simulink model "diff_controller"  (R2024b)
settings: Solver=FixedStepAuto  StartTime=0.0  StopTime=inf  FixedStep=0.001  RelTol=1e-3  EnableMultiTasking=on
InitFcn:
  | Ts = 0.005;
  | diameter = 165; %mm
  | width = 441; %mm
libraries: arduinolib x19, simulink x10, svdutilitieslib x5, simulink_extras x3, arduinosensorlib x2, robotmobilelib x1
(part 2 of 2)

== matlab function diff_controller/Subsystem1/Pose Parser ==
  settings: updateMethod=DISCRETE  sampleTime=Ts
  data: data input; theta output size=[1 1]; distance output size=[1 1]
function [theta, distance] = process_feedback(data)
    % process_feedback searches an array of uint8 values for a valid packet.
    %
    % Packet protocol:
    %   HEADER (uint8)        : 0xAA
    %   THETA (4 x uint8)     : desired theta in rad (stored as 4 bytes)
    %   DISTANCE (4 x uint8)  : desired distance in meter (stored as 4 bytes)
    %   Checksum (uint8)      : XOR checksum of HEADER, THETA, and DISTANCE bytes
    %   Dummy Byte (uint8)    : must equal 0xEE
    %   TERMINATOR (uint8)    : must equal 0xEF
    %
    % If a valid packet is found, the function decodes THETA and DISTANCE;
    % if none is found, it returns the last valid values.
    %
    % The packet is 12 bytes long.
    %

    persistent lastTheta lastDistance;
    if isempty(lastTheta)
        lastTheta = single(0);
    end
    if isempty(lastDistance)
        lastDistance = single(0);
    end

    HEADER   = uint8(170);  % 0xAA
    DUMMY    = uint8(238);  % 0xEE
    TERMINATOR = uint8(239); % 0xEF
    PACKET_SIZE = 12;       

    data = data(:)';

    for i = 1:(length(data) - PACKET_SIZE + 1)
        if data(i) == HEADER
            packet = data(i:(i+PACKET_SIZE-1));

            % Extract fields from the packet:
            % - Byte 1: HEADER (already checked)
            % - Bytes 2-5: THETA bytes
            % - Bytes 6-9: DISTANCE bytes
            % - Byte 10: Checksum
            % - Byte 11: Dummy byte (should equal 0xEE)
            % - Byte 12: Terminator (should equal 0xEF)
            thetaBytes    = packet(2:5);
            distanceBytes = packet(6:9);
            receivedChecksum = packet(10);
            dummy         = packet(11);
            terminator    = packet(12);

            if dummy ~= DUMMY || terminator ~= TERMINATOR
                continue; 
            end
            
            computedChecksum = packet(1);
            for j = 2:9
                computedChecksum = bitxor(computedChecksum, packet(j));
            end

            if computedChecksum ~= receivedChecksum
                continue; 
            end

            theta    = typecast(uint8(thetaBytes), 'single');
            distance = typecast(uint8(distanceBytes), 'single');

            lastTheta = theta;
            lastDistance = distance;
        end
    end

    theta    = lastTheta;
    distance = lastDistance;
   
end

== matlab function diff_controller/Ref Parser/Ref Parser ==
  settings: updateMethod=DISCRETE  sampleTime=Ts
  data: data input; theta output size=[1 1]; distance output size=[1 1]
function [theta, distance] = process_feedback(data)
    % process_feedback searches an array of uint8 values for a valid packet.
    %
    % Packet protocol:
    %   HEADER (uint8)        : 0xAA
    %   THETA (4 x uint8)     : desired theta in rad (stored as 4 bytes)
    %   DISTANCE (4 x uint8)  : desired distance in meter (stored as 4 bytes)
    %   Checksum (uint8)      : XOR checksum of HEADER, THETA, and DISTANCE bytes
    %   Dummy Byte (uint8)    : must equal 0xEE
    %   TERMINATOR (uint8)    : must equal 0xEF
    %
    % If a valid packet is found, the function decodes THETA and DISTANCE;
    % if none is found, it returns the last valid values.
    %
    % The packet is 12 bytes long.
    %

    persistent lastTheta lastDistance;
    if isempty(lastTheta)
        lastTheta = single(0);
    end
    if isempty(lastDistance)
        lastDistance = single(0);
    end

    HEADER   = uint8(170);  % 0xAA
    DUMMY    = uint8(238);  % 0xEE
    TERMINATOR = uint8(239); % 0xEF
    PACKET_SIZE = 12;       

    data = data(:)';

    for i = 1:(length(data) - PACKET_SIZE + 1)
        if data(i) == HEADER
            packet = data(i:(i+PACKET_SIZE-1));

            % Extract fields from the packet:
            % - Byte 1: HEADER (already checked)
            % - Bytes 2-5: THETA bytes
            % - Bytes 6-9: DISTANCE bytes
            % - Byte 10: Checksum
            % - Byte 11: Dummy byte (should equal 0xEE)
            % - Byte 12: Terminator (should equal 0xEF)
            thetaBytes    = packet(2:5);
            distanceBytes = packet(6:9);
            receivedChecksum = packet(10);
            dummy         = packet(11);
            terminator    = packet(12);

            if dummy ~= DUMMY || terminator ~= TERMINATOR
                continue; 
            end
            
            computedChecksum = packet(1);
            for j = 2:9
                computedChecksum = bitxor(computedChecksum, packet(j));
            end

            if computedChecksum ~= receivedChecksum
                continue; 
            end

            theta    = typecast(uint8(thetaBytes), 'single');
            distance = typecast(uint8(distanceBytes), 'single');

            lastTheta = theta;
            lastDistance = distance;
        end
    end

    theta    = lastTheta;
    distance = lastDistance;
   
end

== stateflow chart diff_controller/Chart1 ==
  settings: updateMethod=DISCRETE  sampleTime=Ts
  state Moving
    entry:
    steer_rear = 0;
    speed_rear = 100;
    stear_front = 0;
    speed_front = 0;
    during:
    measured_distance = measured_distance + current_encoder_velocity;
  state Init
    entry:
    steer_rear = 0;
    speed_rear = 0;
    stear_front = 0;
    speed_front = 0;
  state Stopped
    entry:
    steer_rear = 0;
    speed_rear = 0;
    stear_front = 0;
    speed_front = 0;
  state Rotating
    entry:
    steer_rear = 100;
    speed_rear = 0;
    stear_front = -100;
    speed_front = 0;
    during:
    measured_angle = measured_angle + current_angular_velocity;
    exit:
    measured_distance = 0;
    measured_angle = 0;
  (default) -> Init
  Init -> Moving : after(10,sec)
  Stopped -> Moving [order 1] : [measured_distance < set_point]
  Moving -> Stopped : [measured_distance >= set_point]
  Rotating -> Stopped : [measured_angle >= 180]
  Stopped -> Rotating [order 2] : [measured_distance >= set_point]
      | {after(1,sec)}
  data: speed_rear output; current_encoder_velocity input; current_angular_velocity input; set_point input; steer_rear output; measured_distance output =0; speed_front output; stear_front output; measured_angle output =0

== matlab function diff_controller/Encoders/Encoder Parser ==
  settings: updateMethod=DISCRETE  sampleTime=Ts
  data: sample input; rightSpeed output; leftSpeed output
function [rightSpeed, leftSpeed] = encoder_parser(sample)

    persistent rSpeed;
    persistent lSpeed;

    if isempty(rSpeed)
        rSpeed = 0;
        lSpeed = 0;
    end
    headers = find(sample == -21555);
    if diff(headers) == 9
        rSpeed = double(sample(headers(1)+3));
        lSpeed = double(sample(headers(1)+4));
        rightSpeed = -1*rSpeed;
        leftSpeed = lSpeed;
    else
        rightSpeed = -1*rSpeed;
        leftSpeed = lSpeed;
    end
end

== stateflow chart diff_controller/Chart ==
  state Init
    entry:
    steer = 0;
    speed = 0;
  state Moving
    entry:
    steer = 0;
    speed = 100;
  state Rotating
    entry:
    steer = 100;
    speed = 0;
  state Stopped
    entry:
    steer = 0;
    speed = 0;
  (default) -> Init
  Init -> Moving
  Stopped -> Moving [order 1] : [measured_distance < 10 && utrasonic_status == 0]
  Moving -> Stopped : [measured_distance >= 10 || utrasonic_status == 1]
  Rotating -> Stopped : [measured_angle >= 180]
  Stopped -> Rotating [order 2] : [measured_distance >= 10]
  data: utrasonic_status input; measured_distance input; speed output; steer output; measured_angle input

== stateflow chart diff_controller/Chart2 ==
  settings: updateMethod=DISCRETE  sampleTime=Ts
  state Moving
    entry:
    steer_rear = 100;
    speed_rear = 0;
    stear_front =  100;
    speed_front = 0;
    during:
    steer_rear = 100;
    speed_rear = 0;
    stear_front =  100;
    speed_front = 0;
  state Init
    entry:
    steer_rear = 0;
    speed_rear = 0;
    stear_front = 0;
    speed_front = 0;
  (default) -> Init
  Init -> Moving : after(10,sec)
  data: speed_rear output; steer_rear output; speed_front output; stear_front output

== matlab function diff_controller/Encoders1/Encoder Parser ==
  settings: updateMethod=DISCRETE  sampleTime=Ts
  data: sample input; rightSpeed output; leftSpeed output
function [rightSpeed, leftSpeed] = encoder_parser(sample)

    persistent rSpeed;
    persistent lSpeed;

    if isempty(rSpeed)
        rSpeed = 0;
        lSpeed = 0;
    end
    headers = find(sample == -21555);
    if diff(headers) == 9
        rSpeed = double(sample(headers(1)+3));
        lSpeed = double(sample(headers(1)+4));
        rightSpeed = -1*rSpeed;
        leftSpeed = lSpeed;
    else
        rightSpeed = -1*rSpeed;
        leftSpeed = lSpeed;
    end
end

== matlab function diff_controller/Encoders Right/Encoder Parser ==
  settings: updateMethod=DISCRETE  sampleTime=Ts
  data: data input; averageSpeed output
function averageSpeed = process_feedback(data)

% Feedback is sent every 10ms:
% 
% Start frame(unsigned int16) : 0xABCD
% Cmd1(signed int16) : Steer or Brake(hovercar) after normalizing and mixing
% Cmd2(signed int16) : Speed or Throttle(hovercar) after normalizing and mixing
% SpeedR(signed int16) : Measured right wheel speed in RPM
% SpeedL(signed int16) : Measured left wheel speed in RPM
% Battery Voltage(signed int16) : Calibrated Battery Voltage *100
% Temperature(signed int16) : Temperature in °C *10
% Led(unsigned int16) : Used to control the leds on the sideboard
% Checksum(unsigned int16) : XOR checksum
%
%

    persistent lastValidAverageSpeed;

    if isempty(lastValidAverageSpeed)
        lastValidAverageSpeed = int16(0); 
    end
    

    START_FRAME = int16(-21555);
    PACKET_SIZE = 9; 

    data = data(:)';

    for i = 1:(length(data) - PACKET_SIZE + 1)

        if data(i) == START_FRAME
            packet = data(i:(i + PACKET_SIZE - 1));

            Cmd1 = packet(2);
            Cmd2 = packet(3);
            Speed1 = packet(4);
            Speed2 = packet(5);
            BatteryVoltage = packet(6);
            Temperature = packet(7);

            %Note that the original data protocal, the Led is uint16.
            %To solve the data mismatch in the bitxor, we used int16.
            %Original: Led = uint16(packet(8));
            Led = packet(8);
            receivedChecksum = uint16(packet(9));
            
            computedChecksum = bitxor(START_FRAME, Cmd1);
            computedChecksum = bitxor(computedChecksum, Cmd2);
            computedChecksum = bitxor(computedChecksum, Speed1);
            computedChecksum = bitxor(computedChecksum, Speed2);
            computedChecksum = bitxor(computedChecksum, BatteryVoltage);
            computedChecksum = bitxor(computedChecksum, Temperature);
            
            %Data types mismatch. 
            computedChecksum = bitxor(computedChecksum, Led);

            if computedChecksum == receivedChecksum
                lastValidAverageSpeed = int16(mean([(abs(Speed1)), (abs(Speed2))]));
            end
        end
    end

    averageSpeed = lastValidAverageSpeed;
end
